simulink library "ErrorDetector"  (R2016b)
settings: Solver=VariableStepAuto  StartTime=0.0  StopTime=10.0  RelTol=1e-3
undefined symbols (not defined in the file or in its folder): JointControlConfigLHFE, JointControlConfigLKFE, JointControlConfigRHFE, JointControlConfigRKFE
libraries: simulink_extras x8, VariousLibrary x2, EndStopChecker x1, simulink x1, PositionDifferenceChecker x1, TemperaturesJointChecker x1
settings Model: Creator=snyke7  LastModifiedBy=march

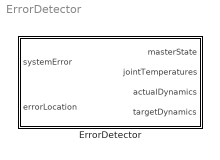
== system ErrorDetector ==
  ErrorDetector : Subsystem

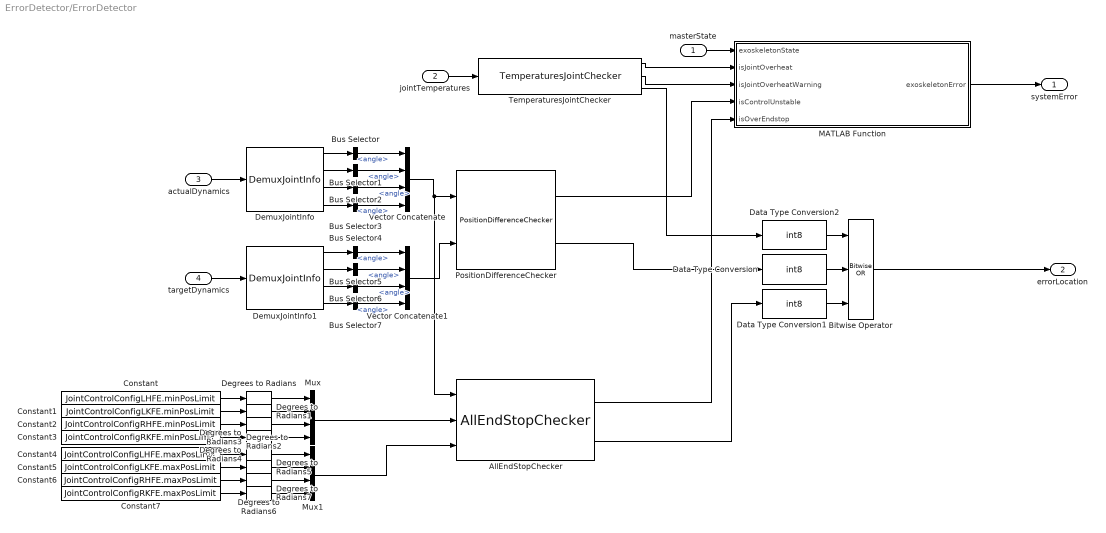
== system ErrorDetector/ErrorDetector ==
  masterState : Inport
  jointTemperatures : Inport  Port=2
  actualDynamics : Inport  Port=3  OutDataTypeStr=Bus: JointDynamics
  targetDynamics : Inport  Port=4  OutDataTypeStr=Bus: JointDynamics
  AllEndStopChecker : EndStopChecker/AllEndStopChecker
  Bitwise Operator : simulink/Logic and Bit Operations/Bitwise Operator  logicop=OR  UseBitMask=off  NumInputPorts=3  BitMask=bin2dec('11011001')  BitMaskRealWorld=Stored Integer
  Bus Selector{,1..7} (8 alike) : BusSelector  OutputSignals=angle
  Constant : Constant  Value=JointControlConfigLHFE.minPosLimit
  Constant1 : Constant  Value=JointControlConfigLKFE.minPosLimit
  Constant2 : Constant  Value=JointControlConfigRHFE.minPosLimit
  Constant3 : Constant  Value=JointControlConfigRKFE.minPosLimit
  Constant4 : Constant  Value=JointControlConfigLHFE.maxPosLimit
  Constant5 : Constant  Value=JointControlConfigLKFE.maxPosLimit
  Constant6 : Constant  Value=JointControlConfigRHFE.maxPosLimit
  Constant7 : Constant  Value=JointControlConfigRKFE.maxPosLimit
  Data Type Conversion : DataTypeConversion  OutDataTypeStr=int8
  Data Type Conversion1 : DataTypeConversion  OutDataTypeStr=int8
  Data Type Conversion2 : DataTypeConversion  OutDataTypeStr=int8
  Degrees to Radians{,1..7} (8 alike) : simulink_extras/Transformations/Degrees to Radians
  DemuxJointInfo : VariousLibrary/DemuxJointInfo
  DemuxJointInfo1 : VariousLibrary/DemuxJointInfo
  MATLAB Function : MATLAB Function  TreatAsAtomicUnit=on
  Mux : Mux
  Mux1 : Mux
  PositionDifferenceChecker : PositionDifferenceChecker/PositionDifferenceChecker
  TemperaturesJointChecker : TemperaturesJointChecker/TemperaturesJointChecker
  Vector Concatenate : Concatenate  NumInputs=4
  Vector Concatenate1 : Concatenate  NumInputs=4
  systemError : Outport  OutDataTypeStr=Enum: ExoskeletonError
  errorLocation : Outport  Port=2
  wires:
  Data Type Conversion2/1 -> Bitwise Operator/1
  TemperaturesJointChecker/3 -> Data Type Conversion2/1
  Data Type Conversion1/1 -> Bitwise Operator/3
  Data Type Conversion/1 -> Bitwise Operator/2
  Bitwise Operator/1 -> errorLocation/1
  AllEndStopChecker/2 -> Data Type Conversion1/1
  PositionDifferenceChecker/2 -> Data Type Conversion/1
  TemperaturesJointChecker/2 -> MATLAB Function/3(isJointOverheatWarning)
  MATLAB Function/1(exoskeletonError) -> systemError/1
  PositionDifferenceChecker/1 -> MATLAB Function/4(isControlUnstable)
  TemperaturesJointChecker/1 -> MATLAB Function/2(isJointOverheat)
  masterState/1 -> MATLAB Function/1(exoskeletonState)
  jointTemperatures/1 -> TemperaturesJointChecker/1
  actualDynamics/1 -> DemuxJointInfo/1
  DemuxJointInfo/1 -> Bus Selector/1
  DemuxJointInfo/2 -> Bus Selector1/1
  DemuxJointInfo/3 -> Bus Selector2/1
  DemuxJointInfo/4 -> Bus Selector3/1
  DemuxJointInfo1/1 -> Bus Selector4/1
  DemuxJointInfo1/2 -> Bus Selector5/1
  DemuxJointInfo1/3 -> Bus Selector6/1
  DemuxJointInfo1/4 -> Bus Selector7/1
  targetDynamics/1 -> DemuxJointInfo1/1
  Bus Selector/1 -> Vector Concatenate/1  "<angle>"
  Bus Selector1/1 -> Vector Concatenate/2  "<angle>"
  Bus Selector2/1 -> Vector Concatenate/3  "<angle>"
  Bus Selector3/1 -> Vector Concatenate/4  "<angle>"
  Bus Selector7/1 -> Vector Concatenate1/4  "<angle>"
  Bus Selector4/1 -> Vector Concatenate1/1  "<angle>"
  Bus Selector6/1 -> Vector Concatenate1/3  "<angle>"
  Bus Selector5/1 -> Vector Concatenate1/2  "<angle>"
  Vector Concatenate/1 -> AllEndStopChecker/1, PositionDifferenceChecker/1
  Vector Concatenate1/1 -> PositionDifferenceChecker/2
  Constant/1 -> Degrees to Radians/1
  Constant1/1 -> Degrees to Radians1/1
  Constant3/1 -> Degrees to Radians3/1
  Constant2/1 -> Degrees to Radians2/1
  Constant4/1 -> Degrees to Radians4/1
  Constant5/1 -> Degrees to Radians5/1
  Constant6/1 -> Degrees to Radians6/1
  Constant7/1 -> Degrees to Radians7/1
  Mux/1 -> AllEndStopChecker/2
  Mux1/1 -> AllEndStopChecker/3
  AllEndStopChecker/1 -> MATLAB Function/5(isOverEndstop)
  Degrees to Radians/1 -> Mux/1
  Degrees to Radians1/1 -> Mux/2
  Degrees to Radians2/1 -> Mux/3
  Degrees to Radians3/1 -> Mux/4
  Degrees to Radians4/1 -> Mux1/1
  Degrees to Radians5/1 -> Mux1/2
  Degrees to Radians6/1 -> Mux1/3
  Degrees to Radians7/1 -> Mux1/4

== matlab function ErrorDetector/MATLAB Function ==
  data: exoskeletonState input; exoskeletonError output; isJointOverheat input; isJointOverheatWarning input; isControlUnstable input; isOverEndstop input
function exoskeletonError = selectErrorWithState(exoskeletonState, isJointOverheat, isJointOverheatWarning, isControlUnstable, isOverEndstop)
% determines exoskeletonError from overheat and unstability flags
% always sends out overheat error, only sends out unstable error if master
% is not in manual state
if(isJointOverheat || isJointOverheatWarning)
    exoskeletonError = ExoskeletonError.EXOSKELETON_JOINT_OVERHEAT;
else
    if(exoskeletonState == ExoskeletonState.FULLMANUAL || exoskeletonState == ExoskeletonState.MANUAL)
        exoskeletonError = ExoskeletonError.EXOSKELETON_NO_ERROR;
    elseif(isOverEndstop)
        exoskeletonError = ExoskeletonError.EXOSKELETON_HARDSTOP_REACHED;
    elseif(isControlUnstable && exoskeletonState ~= ExoskeletonState.SEVERE_ERROR) % when not gaiting, we ignore maxPositionDifference
        exoskeletonError = ExoskeletonError.EXOSKELETON_UNSTABLE_CONTROL;
    else
        exoskeletonError = ExoskeletonError.EXOSKELETON_NO_ERROR;
    end
end
end
